simulink subsystem "Scenario_Command"  (R2025a)
settings: Solver=VariableStepAuto  StartTime=0.0  StopTime=10.0  RelTol=1e-3
settings Model: Creator=Jackt  LastModifiedBy=Jackt

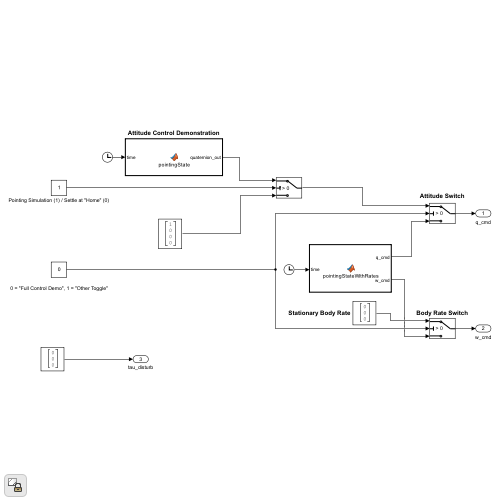
[thumbnail: Simulink's stored preview of the top-level diagram]
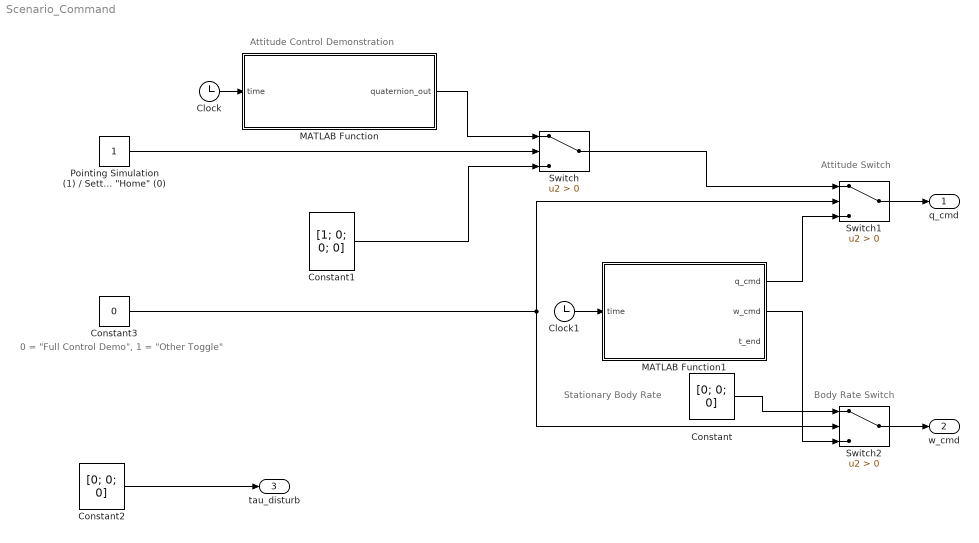
== system Scenario_Command ==
  note: 0 = "Full Control Demo", 1 = "Other Toggle"
  note: Body Rate Switch
  note: Attitude Switch
  note: Attitude Control Demonstration
  note: Stationary Body Rate
  Clock : Clock
  Clock1 : Clock
  Constant : Constant  Value=[0; 0; 0]  VectorParams1D=off
  Constant1 : Constant  Value=[1; 0; 0; 0]  VectorParams1D=off
  Constant2 : Constant  Value=[0; 0; 0]  VectorParams1D=off
  Constant3 : Constant  Value=0
  MATLAB Function : MATLAB Function  TreatAsAtomicUnit=on
  MATLAB Function1 : MATLAB Function  TreatAsAtomicUnit=on
  "Pointing Simulation (1) / Settle at \"Home\" (0)" : Constant
  Switch : Switch  Criteria=u2 > Threshold  SaturateOnIntegerOverflow=off  InputSameDT=off
  Switch1 : Switch  Criteria=u2 > Threshold  SaturateOnIntegerOverflow=off  InputSameDT=off
  Switch2 : Switch  Criteria=u2 > Threshold  SaturateOnIntegerOverflow=off  InputSameDT=off
  q_cmd : Outport
  w_cmd : Outport  Port=2
  tau_disturb : Outport  Port=3
  wires:
  Constant/1 -> Switch2/1
  Constant2/1 -> tau_disturb/1
  Clock/1 -> MATLAB Function/1(time)
  Constant1/1 -> Switch/3
  "Pointing Simulation (1) / Settle at \"Home\" (0)"/1 -> Switch/2
  MATLAB Function/1(quaternion_out) -> Switch/1
  Clock1/1 -> MATLAB Function1/1(time)
  Constant3/1 -> Switch1/2, Switch2/2
  MATLAB Function1/1(q_cmd) -> Switch1/3
  MATLAB Function1/2(w_cmd) -> Switch2/3
  Switch2/1 -> w_cmd/1
  Switch1/1 -> q_cmd/1
  Switch/1 -> Switch1/1

== matlab function Scenario_Command/MATLAB Function1 ==
  data: time input; q_cmd output; w_cmd output; t_end output
function [q_cmd, w_cmd, t_end] = pointingStateWithRates(time)
%POINTINGSTATEWITHRATES Quaternion + body-rate command.
% Per attitude:
%   1) Point and settle
%   2) Spin forward
%   3) Spin backward
%   4) Settle
% Then move to the next attitude.
% After C, return home and hold.
%
% Scalar-first quaternions: [qw; qx; qy; qz]
% Body rates in rad/s, expressed in the body frame of the commanded attitude.

% --- Setpoints (base attitudes) ---
q_home = [1; 0; 0; 0];
q_A    = [0.70710678; 0.70710678; 0; 0]; % +90 deg about X
q_B    = [0.70710678; 0; 0.70710678; 0]; % +90 deg about Y
q_C    = [0.70710678; 0; 0; 0.70710678]; % +90 deg about Z

% --- Timing (seconds) ---
T_settle1 = 10;  % settle after moving to base attitude
T_spin    = 5;   % spin forward
T_flip    = 5;   % spin backward
T_settle2 = 5;  % settle after finishing the spin pair
T_block   = T_settle1 + T_spin + T_flip + T_settle2;

T_home_final = 15; % final home hold

% --- Spin speed (rad/s) ---
spin_deg_s = 45;
w_mag = deg2rad(spin_deg_s);

% Total sim time you should run to
t_end = 3*T_block + T_home_final;

% --- Defaults ---
q_cmd = q_home;
w_cmd = [0; 0; 0];

% --- Select which base attitude block we are in ---
if time < 1*T_block
    q_base = q_A;
    axis_body = [0; 0; 1];   % spin about body Z while at A
    t_local = time;
elseif time < 2*T_block
    q_base = q_B;
    axis_body = [1; 0; 0];   % spin about body X while at B
    t_local = time - 1*T_block;
elseif time < 3*T_block
    q_base = q_C;
    axis_body = [0; 1; 0];   % spin about body Y while at C
    t_local = time - 2*T_block;
elseif time < t_end
    q_cmd = q_home;
    w_cmd = [0; 0; 0];
    q_cmd = q_cmd / max(norm(q_cmd), 1e-12);
    return;
else
    q_cmd = q_home;
    w_cmd = [0; 0; 0];
    q_cmd = q_cmd / max(norm(q_cmd), 1e-12);
    return;
end

% --- Within a block: settle1, spin forward, spin backward, settle2 ---
if t_local < T_settle1
    q_spin = [1; 0; 0; 0];
    w_cmd  = [0; 0; 0];

elseif t_local < (T_settle1 + T_spin)
    t_spin = t_local - T_settle1;
    theta  = w_mag * t_spin;
    q_spin = axisAngleToQuat(axis_body, theta);
    w_cmd  = w_mag * axis_body;

elseif t_local < (T_settle1 + T_spin + T_flip)
    t_rev  = t_local - (T_settle1 + T_spin);
    theta0 = w_mag * T_spin;
    theta  = theta0 - w_mag * t_rev;
    q_spin = axisAngleToQuat(axis_body, theta);
    w_cmd  = -w_mag * axis_body;

else
    q_spin = [1; 0; 0; 0];
    w_cmd  = [0; 0; 0];
end

% --- Compose commanded attitude: base then spin ---
q_cmd = quatMultiplySF(q_base, q_spin);
q_cmd = q_cmd / max(norm(q_cmd), 1e-12);

end

% ===================== Helpers =====================

function q = axisAngleToQuat(axis_body, theta)
axis_body = axis_body / max(norm(axis_body), 1e-12);
half = 0.5 * theta;
q = [cos(half); axis_body * sin(half)];
q = q / max(norm(q), 1e-12);
end

function q = quatMultiplySF(q1, q2)
w1 = q1(1); v1 = q1(2:4);
w2 = q2(1); v2 = q2(2:4);

w = w1*w2 - dot(v1, v2);
v = w1*v2 + w2*v1 + cross(v1, v2);

q = [w; v];
q = q / max(norm(q), 1e-12);
end

== matlab function Scenario_Command/MATLAB Function ==
  data: quaternion_out output; time input
function quaternion_out = pointingState(time)
%POINTINGSTATE Simple attitude sequence:
%home -> +90deg about X -> +90deg about Y -> +90deg about Z -> home

%Setpoints
q_home = [1; 0; 0; 0];
q_x90  = [0.70710678; 0.70710678; 0; 0];
q_y90  = [0.70710678; 0; 0.70710678; 0];
q_z90  = [0.70710678; 0; 0; 0.70710678];

%Timing
Thold = 15; % seconds per state

%Piecewise command
if time < 1*Thold
    q_cmd = q_home;
elseif time < 2*Thold
    q_cmd = q_x90;
elseif time < 3*Thold
    q_cmd = q_y90;
elseif time < 4*Thold
    q_cmd = q_z90;
else
    q_cmd = q_home;
end

%Normalize output
quaternion_out = q_cmd / norm(q_cmd);

end
